simulink model "ex_bus_ports"  (R2019b)
settings: Solver=VariableStepAuto  StartTime=0.0  StopTime=10.0  RelTol=1e-3
settings Model: Creator=The MathWorks, Inc.  LastModifiedBy=bhisma
settings DebuggingCC: PregeneratedLibrarySubsystemCodeDiagnostic=none  ArithmeticOperatorsInVariantConditions=warning
settings SFSimCC: SimUseLocalCustomCode=off  CustomCodeUndefinedFunction=UseInterfaceOnly
settings RTWCC: RTWUseLocalCustomCode=off
settings CodeAppCC: StateflowObjectComments=on

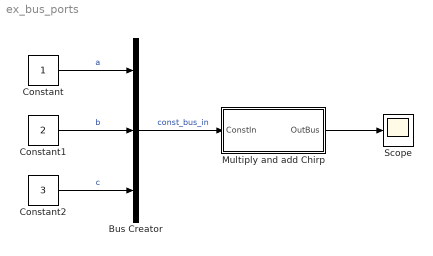
== system ex_bus_ports ==
  Bus Creator : BusCreator  Inputs=3
  Constant : Constant
  Constant1 : Constant  Value=2
  Constant2 : Constant  Value=3
  Multiply and add Chirp : Subsystem
  Scope : Scope
  wires:
  Constant/1 -> Bus Creator/1  "a"
  Constant1/1 -> Bus Creator/2  "b"
  Constant2/1 -> Bus Creator/3  "c"
  Bus Creator/1 -> Multiply and add Chirp/1(ConstIn)  "const_bus_in"
  Multiply and add Chirp/1(OutBus) -> Scope/1

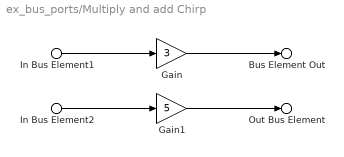
== system ex_bus_ports/Multiply and add Chirp ==
  In Bus Element1 : Inport  PortName=ConstIn  Element=a
  In Bus Element2 : Inport  PortName=ConstIn  Element=b
  Gain : Gain  Gain=3
  Gain1 : Gain  Gain=5
  Bus Element Out : Outport  VectorParamsAs1DForOutWhenUnconnected=off  PortName=OutBus  Element=a*3
  Out Bus Element : Outport  VectorParamsAs1DForOutWhenUnconnected=off  PortName=OutBus  Element=b*5
  wires:
  In Bus Element2/1 -> Gain1/1
  Gain/1 -> Bus Element Out/1
  Gain1/1 -> Out Bus Element/1
  In Bus Element1/1 -> Gain/1
